simulink model "Expt2"  (R2020b)
settings: Solver=VariableStepAuto  StartTime=0.0  StopTime=0.5  RelTol=1e-3
settings Model: Creator=geniu  LastModifiedBy=geniu

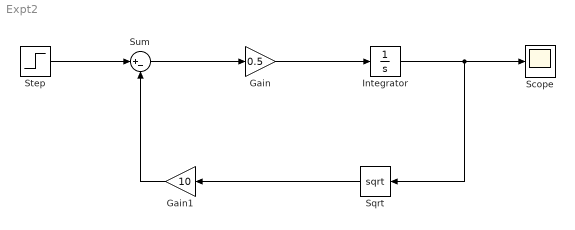
== system Expt2 ==
  Gain : Gain  Gain=0.5
  Gain1 : Gain  Gain=10
  Integrator : Integrator
  Scope : Scope
  Sqrt : Sqrt  SaturateOnIntegerOverflow=on
  Step : Step  Time=0  SampleTime=0
  Sum : Sum  Inputs=|+-
  wires:
  Step/1 -> Sum/1
  Sum/1 -> Gain/1
  Gain/1 -> Integrator/1
  Integrator/1 -> Sqrt/1, Scope/1
  Gain1/1 -> Sum/2
  Sqrt/1 -> Gain1/1
